simulink model "nanorobot_non_lineare"  (R2018a)
settings: Solver=VariableStepAuto  StartTime=0.0  StopTime=10  RelTol=1e-3
undefined symbols (not defined in the file): dati, input
settings Model: Creator=Ivonne  LastModifiedBy=Ivonne

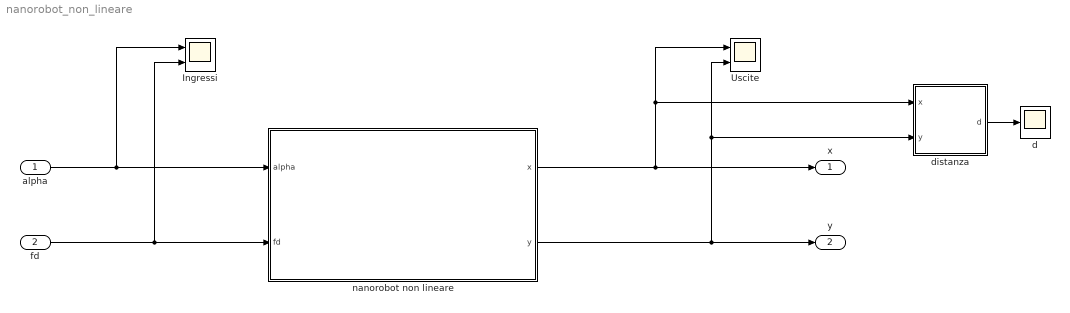
== system nanorobot_non_lineare ==
  alpha : Inport
  fd : Inport  Port=2
  Ingressi : Scope  NumInputPorts=2
  Uscite : Scope  NumInputPorts=2
  d : Scope
  "distanza " : Subsystem
  nanorobot non lineare : Subsystem
  x : Outport
  y : Outport  Port=2
  wires:
  alpha/1 -> nanorobot non lineare/1(alpha), Ingressi/1
  nanorobot non lineare/1(x) -> x/1, Uscite/1, "distanza "/1(x)
  nanorobot non lineare/2(y) -> y/1, Uscite/2, "distanza "/2(y)
  "distanza "/1(d) -> d/1
  fd/1 -> Ingressi/2, nanorobot non lineare/2(fd)

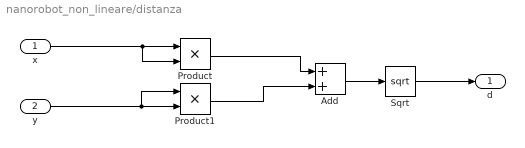
== system nanorobot_non_lineare/distanza  ==
  x : Inport
  y : Inport  Port=2
  Add : Sum
  Product : Product
  Product1 : Product
  Sqrt : Sqrt  OutputSignalType=real  SaturateOnIntegerOverflow=on
  d : Outport
  wires:
  Add/1 -> Sqrt/1
  Sqrt/1 -> d/1
  y/1 -> Product1/1, Product1/2
  x/1 -> Product/1, Product/2
  Product/1 -> Add/1
  Product1/1 -> Add/2

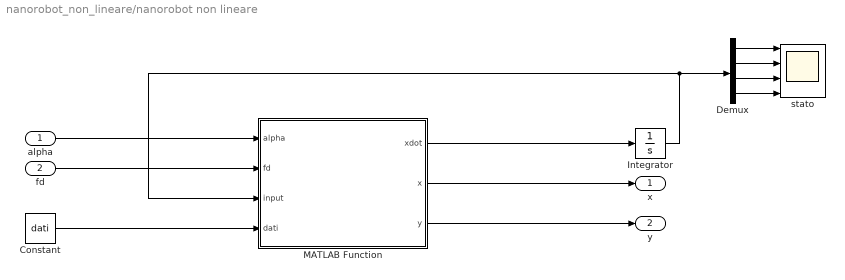
== system nanorobot_non_lineare/nanorobot non lineare ==
  alpha : Inport
  fd : Inport  Port=2
  Constant : Constant  Value=dati
  Demux : Demux
  Integrator : Integrator  InitialCondition=input
  MATLAB Function : MATLAB Function  TreatAsAtomicUnit=on
  stato : Scope  NumInputPorts=4
  x : Outport
  y : Outport  Port=2
  wires:
  MATLAB Function/1(xdot) -> Integrator/1
  Integrator/1 -> MATLAB Function/3(input), Demux/1
  MATLAB Function/2(x) -> x/1
  Constant/1 -> MATLAB Function/4(dati)
  Demux/1 -> stato/1
  Demux/2 -> stato/2
  Demux/3 -> stato/3
  Demux/4 -> stato/4
  MATLAB Function/3(y) -> y/1
  fd/1 -> MATLAB Function/2(fd)
  alpha/1 -> MATLAB Function/1(alpha)

== matlab function nanorobot_non_lineare/nanorobot non lineare/MATLAB Function ==
  data: xdot output; alpha input; fd input; input input; x output; dati input; y output
function [ xdot, x, y ] = fcn(alpha, fd, input, dati)
% input : condizioni iniziali
% u : ingresso del sistema -> [ alpha, fd]
% dati : parametri del modello fisico -> [ R, Fm, m, eta,l, dP, r, vf ]
R= dati(1);                 
Fm = dati(2);  
m = dati(3);
eta = dati(4);
l = dati(5);
dP = dati(6);
r = dati(7);
vf = dati(8);
% variabili di stato 
% x1 = x, x2 = xp -> x1p, x3 = y, x4 = yp -> x3p
% allora xpp = x2p e ypp = x4p
x1 = input(1); % xdot(1) = x2 -> 1/s 
x2 = input(2); % xdot(2) = x2p -> 1/s 
x3 = input(3); % xdot(3) = x4 -> 1/s
x4 = input(4); % xdot(4) = x4p -> 1/s
% forma di stato
xdot = [ x2;
         ((-6*pi*eta*R)/m)*x2 + ((6*pi*eta*R)/m)*vf + (Fm/m)*cos(alpha) + fd/m;
         x4;
         ((-6*pi*eta*R)/m)*x4 + (Fm/m)*sin(alpha)];

% coordinate cartesiane
x = x1;
y = x3;
